simulink model "csws_simulink_model"  (R2021a)
settings: Solver=FixedStepAuto  StartTime=0.0  StopTime=15  RelTol=1e-3
model workspace (MAT data in the model file):
  t = 0
libraries: simulink x1
(part 1 of 2)
settings Model: Creator=Martin  LastModifiedBy=Martin
settings SolverCC: AutoInsertRateTranBlk=on

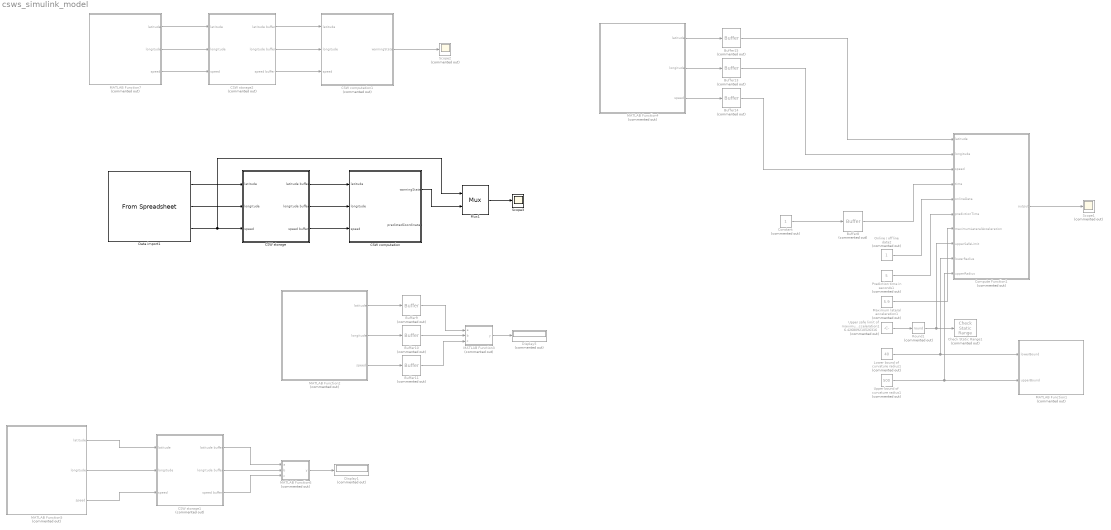
== system csws_simulink_model ==
  Buffer{8..11,13..15} (7 alike) : Buffer  Commented=on  N=3  V=2  ic=-199  OutputFrames=off
  CSW computation : MATLAB Function  TreatAsAtomicUnit=on  mask{timeRate=1, predictionTime=5, maximumLateralAcceleration=5.9, upperSafeLimit=70, lowerRadius=0, upperRadius=5000, visualizeTrajectory=on}
      mask prompts: timeRate "Time frequency of input data (s)"; predictionTime "Prediction time (s)"; maximumLateralAcceleration "Maximum lateral acceleration (m/s^2)"; upperSafeLimit "Safe limit to decrease value of lateral acceleration (0-100%)"; lowerRadius "Lower limit (m)"; upperRadius "Upper limit (m)"; visualizeTrajectory "Visualize trajectory"
  CSW computation1 : MATLAB Function  Commented=on  TreatAsAtomicUnit=on  mask{timeRate=1, predictionTime=5, maximumLateralAcceleration=5.9, upperSafeLimit=70, lowerRadius=0, upperRadius=5000, visualizeTrajectory=on}
      mask prompts: timeRate "Time frequency of input data (s)"; predictionTime "Prediction time (s)"; maximumLateralAcceleration "Maximum lateral acceleration (m/s^2)"; upperSafeLimit "Safe limit to decrease value of lateral acceleration (0-100%)"; lowerRadius "Lower limit (m)"; upperRadius "Upper limit (m)"; visualizeTrajectory "Visualize trajectory"
  CSW storage : Subsystem
  CSW storage1 : Subsystem  Commented=on
  CSW storage2 : Subsystem  Commented=on
  Check Static Range1 : simulink/Model Verification/Check  Static Range  Description=0 <= u <= 100  Commented=on  max=100  max_included=on  min=0  min_included=on  enabled=on  stopWhenAssertionFail=on  export=off  icon=graphic
      settings: SourceProductBaseCode=SL
  Compute Function1 : MATLAB Function  Commented=on  TreatAsAtomicUnit=on
  Constant : Constant  Commented=on
  Data import1 : FromSpreadsheet  FileName=C:\Users\Martin\MATLAB\Projects\curve-speed-warning-system\src\exampleData2.xlsx  SheetName=Hárok1  Range=A1:C11  TreatFirstColumnAs=Data  SampleTime=-1  OutputAfterLastPoint=Ground value
  Display1 : Display  Commented=on
  Display5 : Display  Commented=on
  Lower bound of curvature radius1 : Constant  Commented=on  Value=40
  MATLAB Function1 : MATLAB Function  Commented=on  TreatAsAtomicUnit=on
  MATLAB Function2 : MATLAB Function  Commented=on  TreatAsAtomicUnit=on  mask{inputPort=15}
      mask prompts: inputPort "Serial port - COM"
  MATLAB Function3 : MATLAB Function  Commented=on  TreatAsAtomicUnit=on
  MATLAB Function4 : MATLAB Function  Commented=on  TreatAsAtomicUnit=on
  MATLAB Function5 : MATLAB Function  Commented=on  TreatAsAtomicUnit=on  mask{inputPort=15}
      mask prompts: inputPort "Serial port - COM"
  MATLAB Function6 : MATLAB Function  Commented=on  TreatAsAtomicUnit=on
  MATLAB Function7 : MATLAB Function  Commented=on  TreatAsAtomicUnit=on  mask{inputPort=15}
      mask prompts: inputPort "Serial port - COM"
  Maximum lateral acceleration1 : Constant  Commented=on  Value=5.9
  Mux1 : Mux  Inputs=2
  Online / offline data2 : Constant  Commented=on
  Prediction time in seconds1 : Constant  Commented=on  Value=5
  Round1 : Rounding  Commented=on  Operator=round
  Scope1 : Scope  Commented=on
  Scope2 : Scope  Commented=on
  Scope3 : Scope
  Upper bound of curvature radius1 : Constant  Commented=on  Value=500
  Upper safe limit of maximum lateral acceleration1 : Constant  Commented=on  Value=6.426809210526316
  wires:
  Buffer8/1 -> Compute Function1/4(time)
  Compute Function1/1(output) -> Scope1/1
  Prediction time in seconds1/1 -> Compute Function1/6(predictionTime)
  Upper bound of curvature radius1/1 -> MATLAB Function1/2(upperBound), Compute Function1/10(upperRadius)
  Upper safe limit of maximum lateral acceleration1/1 -> Round1/1
  Lower bound of curvature radius1/1 -> MATLAB Function1/1(lowerBound), Compute Function1/9(lowerRadius)
  Round1/1 -> Check Static Range1/1, Compute Function1/8(upperSafeLimit)
  Maximum lateral acceleration1/1 -> Compute Function1/7(maximumLateralAcceleration)
  Online / offline data2/1 -> Compute Function1/5(onlineData)
  MATLAB Function2/1(latitude) -> Buffer9/1
  MATLAB Function2/2(longitude) -> Buffer10/1
  MATLAB Function2/3(speed) -> Buffer11/1
  Buffer9/1 -> MATLAB Function3/1(a)
  Buffer11/1 -> MATLAB Function3/3(c)
  Buffer10/1 -> MATLAB Function3/2(b)
  MATLAB Function3/1(y) -> Display5/1
  MATLAB Function4/2(longitude) -> Buffer13/1
  MATLAB Function4/3(speed) -> Buffer14/1
  MATLAB Function4/1(latitude) -> Buffer15/1
  Buffer15/1 -> Compute Function1/1(latitude)
  Buffer13/1 -> Compute Function1/2(longitude)
  Buffer14/1 -> Compute Function1/3(speed)
  Constant/1 -> Buffer8/1
  Mux1/1 -> Scope3/1
  Data import1/3 -> Mux1/1, CSW storage/3(speed)
  CSW computation/1(warningState) -> Mux1/2
  Data import1/1 -> CSW storage/1(latitude)
  Data import1/2 -> CSW storage/2(longitude)
  CSW storage/1(latitude buffer) -> CSW computation/1(latitude)
  CSW storage/2(longitude buffer) -> CSW computation/2(longitude)
  CSW storage/3(speed buffer) -> CSW computation/3(speed)
  MATLAB Function6/1(y) -> Display1/1
  MATLAB Function5/2(longitude) -> CSW storage1/2(longitude)
  CSW storage1/2(longitude buffer) -> MATLAB Function6/2(b)
  CSW storage1/1(latitude buffer) -> MATLAB Function6/1(a)
  CSW storage1/3(speed buffer) -> MATLAB Function6/3(c)
  MATLAB Function5/1(latitude) -> CSW storage1/1(latitude)
  MATLAB Function5/3(speed) -> CSW storage1/3(speed)
  MATLAB Function7/3(speed) -> CSW storage2/3(speed)
  MATLAB Function7/2(longitude) -> CSW storage2/2(longitude)
  MATLAB Function7/1(latitude) -> CSW storage2/1(latitude)
  CSW storage2/1(latitude buffer) -> CSW computation1/1(latitude)
  CSW storage2/2(longitude buffer) -> CSW computation1/2(longitude)
  CSW storage2/3(speed buffer) -> CSW computation1/3(speed)
  CSW computation1/1(warningState) -> Scope2/1

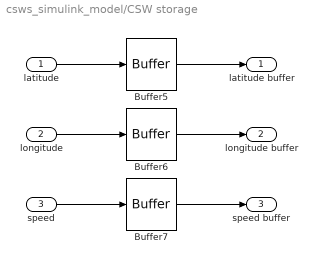
== system csws_simulink_model/CSW storage ==
  latitude : Inport
  longitude : Inport  Port=2
  speed : Inport  Port=3
  Buffer5 : Buffer  N=3  V=2  ic=-199  OutputFrames=off
  Buffer6 : Buffer  N=3  V=2  ic=-199  OutputFrames=off
  Buffer7 : Buffer  N=3  V=2  ic=-199  OutputFrames=off
  latitude buffer : Outport
  longitude buffer : Outport  Port=2
  speed buffer : Outport  Port=3
  wires:
  speed/1 -> Buffer7/1
  Buffer5/1 -> latitude buffer/1
  longitude/1 -> Buffer6/1
  Buffer7/1 -> speed buffer/1
  Buffer6/1 -> longitude buffer/1
  latitude/1 -> Buffer5/1

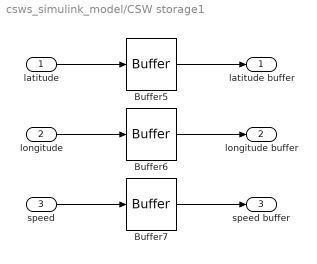
== system csws_simulink_model/CSW storage1 ==
  latitude : Inport
  longitude : Inport  Port=2
  speed : Inport  Port=3
  Buffer5 : Buffer  N=3  V=2  ic=-199  OutputFrames=off
  Buffer6 : Buffer  N=3  V=2  ic=-199  OutputFrames=off
  Buffer7 : Buffer  N=3  V=2  ic=-199  OutputFrames=off
  latitude buffer : Outport
  longitude buffer : Outport  Port=2
  speed buffer : Outport  Port=3
  wires:
  speed/1 -> Buffer7/1
  Buffer5/1 -> latitude buffer/1
  longitude/1 -> Buffer6/1
  Buffer7/1 -> speed buffer/1
  Buffer6/1 -> longitude buffer/1
  latitude/1 -> Buffer5/1

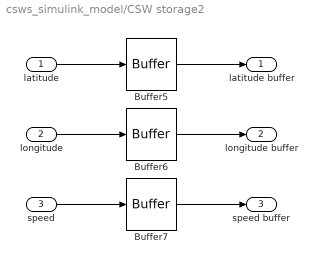
== system csws_simulink_model/CSW storage2 ==
  latitude : Inport
  longitude : Inport  Port=2
  speed : Inport  Port=3
  Buffer5 : Buffer  N=3  V=2  ic=-199  OutputFrames=off
  Buffer6 : Buffer  N=3  V=2  ic=-199  OutputFrames=off
  Buffer7 : Buffer  N=3  V=2  ic=-199  OutputFrames=off
  latitude buffer : Outport
  longitude buffer : Outport  Port=2
  speed buffer : Outport  Port=3
  wires:
  speed/1 -> Buffer7/1
  Buffer5/1 -> latitude buffer/1
  longitude/1 -> Buffer6/1
  Buffer7/1 -> speed buffer/1
  Buffer6/1 -> longitude buffer/1
  latitude/1 -> Buffer5/1

== matlab function csws_simulink_model/CSW computation1 ==
  data: latitude input; longitude input; warningState output; speed input
function warningState = CSW(latitude,longitude,speed)

    coder.extrinsic('plot');
    coder.extrinsic('legend');
    coder.extrinsic('audioread');
    coder.extrinsic('audioplayer');
    coder.extrinsic('serialport');
    coder.extrinsic('readline');
    coder.extrinsic('nmeaParser');
    coder.extrinsic('getfield');
    coder.extrinsic('set_param');
    coder.extrinsic('ceil');
    coder.extrinsic('str2double');
    coder.extrinsic('get_param');
    coder.extrinsic('gcb');
    
    predictionTime = double(0);
    predictionTime = str2double(get_param(gcb,'predictionTime'));
    maximumLateralAcceleration = double(0);
    maximumLateralAcceleration = str2double(get_param(gcb,'maximumLateralAcceleration'));
    upperSafeLimit = double(0);
    upperSafeLimit = str2double(get_param(gcb,'upperSafeLimit'));
    lowerRadius = double(0);
    lowerRadius = str2double(get_param(gcb,'lowerRadius'));
    upperRadius = double(0);
    upperRadius = str2double(get_param(gcb,'upperRadius'));
    timeRate = double(0);
    timeRate = str2double(get_param(gcb,'timeRate'));
    visualizeTrajectory = str2bool(get_param(gcb,'visualizeTrajectory'));
    
    if(upperSafeLimit > 100 || upperSafeLimit < 0)
        error('Invalid value of safe limit, set value in range 0 to 100')
    end
    
    if(lowerRadius < 0 || upperRadius < 0)
        error('Negative value of curvature bound is not supported')
    end

    if(lowerRadius > upperRadius)
        error('Lower bound of curvature radius must be smaller than upper bound')
    end
    
    if(upperSafeLimit > 100 || upperSafeLimit < 0)
        error('Negative value of time frequency is not supported')
    end

%     coder.varsize('output');

    [y, Fs] = audioread('alert.mp3');
    player = audioplayer(y, Fs);
    
    index = 3;

    data = [latitude(:) longitude(:) speed(:)];

    if ismember(-199, data)
        warningState = 0;
        return;
    end

    if (ismember(0, latitude(:)) && ismember(0, longitude(:)) && ismember(0, speed(:)))
        error('Input data contains an invalid zero value/s')
    end

    data = centerDataArray(data);

    allData = [data(index - 2,1) data(index - 2,2) data(index - 2,3); 
        data(index - 1,1) data(index - 1,2) data(index - 1,3); 
        data(index,1) data(index,2) data(index,3)
        ];
    predictedData = [data(index,1) data(index,2) data(index,3)];

    temp_data = [
        data(length(data(:,1))-2,1) data(length(data(:,1))-2,2) data(length(data(:,1))-2,3);
        data(length(data(:,1))-1,1) data(length(data(:,1))-1,2) data(length(data(:,1))-1,3); 
        data(length(data(:,1)),1) data(length(data(:,1)),2) data(length(data(:,1)),3)
        ];

    steps = 0;
    steps = ceil(predictionTime / timeRate);

    for time = 1:steps
        [predictedX, predictedY] = predictCoordinates(temp_data, 3, timeRate);  

        temp_data = [temp_data(2,1) temp_data(2,2) temp_data(2,3);
            temp_data(3,1) temp_data(3,2) temp_data(3,3);
            predictedX predictedY getNextSpeed(temp_data, 3);
            ];

        allData = [allData; [temp_data(3,1) temp_data(3,2) temp_data(3,3)]];
        predictedData = [predictedData; [temp_data(3,1) temp_data(3,2) temp_data(3,3)]];
    end

    allData = computeCurvatureRadiusAndSpeed(allData,maximumLateralAcceleration*((100-upperSafeLimit)/100));

    N = size(allData,1);
    allData = [allData,zeros(N,1)];

    allData = checkCurvatureRadiusAndSpeed(allData, lowerRadius, upperRadius);

    if ismember(1, allData(7,:))
        warningState = 1;
    else
        warningState = 0;
    end

    if(visualizeTrajectory)
        plotOutput(allData, predictedData, timeRate, player);
    end
%     else
% %         set_param('asik','Commented','on')
% %         PORT = "COM15";
%         PORT = serialPort;
%         device = serialport(PORT,9600)
%         pnmea = nmeaParser("MessageIDs", "RMC");
%         
%         record = readline(device);
%         
%         while (isempty(record) || ~startsWith(record,'$GPRMC'))
%             record = readline(device);
%         end        
%         
%         nvm = pnmea(record);
%         Latitude = getfield(nvm,'Latitude');
%         Longitude = getfield(nvm,'Longitude');
%         Speed = getfield(nvm,'GroundSpeed');
%         Time = getfield(nvm,'UTCDateTime');
% %         fldnm = 'Status';
% %         nx2 = nvm.parameters.(fldnm)
% %         latit = output(Latitude)
% %         gpsData = struct('Latitude',output.Latitude,'Longitude',output.Longitude,'Speed',output.GroundSpeed,'Time',output.UTCDateTime,'Status',output.Status);
% 
% 
% %     if (speed(3) > 21)
% %         output = 1
% %     else
% %         output = 0
% %     end
% 
% 
%         warningState = 3
%     end

end

function MyBeep()
    coder.extrinsic('audioplayer');
    coder.extrinsic('play');
    persistent AP
    Play_Data = ([sin(1:.6:400), sin(1:.7:400), sin(1:.4:400)]);
    AP = audioplayer(Play_Data(:), 22050);
    play(AP);
end

function [output]=str2bool(string)
   if strcmp(string,'off')
     output = false;
   else
     output = true;
   end
end

%% plot output prediction trajectory with / without warning

function plotOutput(allData, predictedData, timeRate, player)
    coder.extrinsic('plot');
    coder.extrinsic('legend');
    coder.extrinsic('playblocking');
    coder.extrinsic('play');
    coder.extrinsic('strcat');
    
    x_min = min(allData(:,1)) - 5;
    x_max = max(allData(:,1)) + 5;
    
    x1 =  abs(x_min);
    x2 =  abs(x_max);
    
    result = x1;
    if(x1 < x2)
        result = x2;
    end
    
    y_min = min(allData(:,2)) - 5;
    y_max = max(allData(:,2)) + 5;
    
    plot(allData(:,1), allData(:,2), 'b-o', 'DisplayName','referenced coordinates')
    xlim([-result result])
    ylim([y_min y_max])
    hold on
    plot(predictedData(:,1), predictedData(:,2), 'g-o', 'DisplayName','predicted coordinates')
    plot(predictedData(1,1), predictedData(1,2), 'k-o', 'DisplayName','actual position')
    title(sprintf('point frequency is %.1f second/s',timeRate));
    legend('referenced coordinates','predicted coordinates','actual position')
    
    if ismember(1, allData(:,7))
        set(gca, 'Color',[1 0 0])
%         MyBeep()
%         playblocking(player); 
    else
        set(gca, 'Color',[1 1 1])
    end

    hold off
end

%% compute radius of curvature and recommended speed

function [predictedData] = computeCurvatureRadiusAndSpeed(predictedData,safeLimitOfLateralAcceleration)
    Alateral_max = safeLimitOfLateralAcceleration;

    [pathdistance,R,~] = curvature([predictedData(:,1) predictedData(:,2)]);
    predictedData = [predictedData pathdistance R];
    predictedData = [predictedData sqrt(predictedData(:, 5) * Alateral_max)];
end


%% reference to: https://uk.mathworks.com/matlabcentral/fileexchange/69452-curvature-of-a-1d-curve-in-a-2d-or-3d-space 

function [L,R,k] = curvature(input)
% Radius of curvature and curvature vector for 2D or 3D curve
%  [L,R,k] = curvature(X)
%   X:   2 or 3 column array of x, y (and possibly z) coordiates
%   L:   Cumulative arc length
%   R:   Radius of curvature
%   k:   Curvature vector
% The scalar curvature value is 1./R
% Version 2.6: Calculates end point values for closed curve
%   fefefe = X

  coder.varsize('X');
  coder.varsize('L');
  coder.varsize('R');
  coder.varsize('k');
  X = input;

  N = size(X,1);
  dims = size(X,2);
  if dims == 2
    X = [X,zeros(N,1)];  % Use 3D expressions for 2D as well
  end
  L = zeros(N,1);
  R = NaN(N,1);
  k = NaN(N,3);
  for i = 2:N-1
    [R(i),~,k(i,:)] = circumcenter(X(i,:)',X(i-1,:)',X(i+1,:)');
    L(i) = L(i-1)+norm(X(i,:)-X(i-1,:));
  end
  if norm(X(1,:)-X(end,:)) < 1e-10 % Closed curve. 
    [R(1),~,k(1,:)] = circumcenter(X(end-1,:)',X(1,:)',X(2,:)');
    R(end) = R(1);
    k(end,:) = k(1,:);
    L(end) = L(end-1) + norm(X(end,:)-X(end-1,:));
  end
  i = N;
  L(i) = L(i-1)+norm(X(i,:)-X(i-1,:));
  if dims == 2
    k = k(:,1:2);
  end
end

%% reference to: https://uk.mathworks.com/matlabcentral/fileexchange/69452-curvature-of-a-1d-curve-in-a-2d-or-3d-space 

function [R,M,k] = circumcenter(A,B,C)
% Center and radius of the circumscribed circle for the triangle ABC
%  A,B,C  3D coordinate vectors for the triangle corners
%  R      Radius
%  M      3D coordinate vector for the center
%  k      Vector of length 1/R in the direction from A towards M
%         (Curvature vector)
  D = cross(B-A,C-A);
  b = norm(A-C);
  c = norm(A-B);
  if nargout == 1
    a = norm(B-C);     % slightly faster if only R is required
    R = a*b*c/2/norm(D);
    if norm(D) == 0
      R = Inf;
    end
    return
  end
  E = cross(D,B-A);
  F = cross(D,C-A); 
  G = (b^2*E-c^2*F)/norm(D)^2/2;
  M = A + G;
  R = norm(G);  % Radius of curvature
  if R == 0
    k = G;
  elseif norm(D) == 0
    R = Inf;
    k = D;
  else
    k = G'/R^2;   % Curvature vector
  end
end

%% check if radius of curvature is valid and actual speed is higher than recommended

function [predictedData] = checkCurvatureRadiusAndSpeed(predictedData,lowerRadius,upperRadius)
    Rmin = lowerRadius;
    Rmax = upperRadius;
    
    for k=1:size(predictedData,1)
        if predictedData(k,5) < Rmin || predictedData(k,5) > Rmax
            predictedData(k,7) = 0;
        else
            if predictedData(k,3) > predictedData(k,6)
                predictedData(k,7) = 1;
            else
                predictedData(k,7) = 0;
            end
        end
    end
end

%% compute angle between coordinates

function next_angle = computeCoordinateAngle(data, index, time)
    prev_angle = atan2( (data(index - 1,2) - data(index - 2,2)) , (data(index - 1,1) - data(index - 2,1)));
    act_angle = atan2( (data(index,2) - data(index - 1,2)) , (data(index,1) - data(index - 1,1)));
    
    next_angle = act_angle + time*(act_angle - prev_angle);
end

%% convert latitude, longitude to cartesian coordinate system

function [data] = centerDataArray(data)
    centered_point = [0 1];
    
    data = convertDataArray(data);

    angle = atan2(centered_point(1,2) - data(3,2), centered_point(1,1) - data(3,1)) - atan2(data(2,2) - data(3,2), data(2,1) - data(3,1));
    result = deg2rad(180) - angle;

    x2 = data(2,1) * cos(result) + data(2,2) * sin(result);
    y2 = data(2,1) * -sin(result) + data(2,2) *  cos(result);

    x1 = data(1,1) * cos(result) + data(1,2) * sin(result);
    y1 = data(1,1) * -sin(result) + data(1,2) *  cos(result);

    centeredData = [x1 y1; x2 y2; data(3,1) data(3,2)];
    data(:,1) = centeredData(:,1);
    data(:,2) = centeredData(:,2);
end

%% convert latitude, longitude to cartesian coordinate system

function [data] = convertDataArray(data)
    coder.extrinsic('latlon2local');
    [xCoordinate, yCoordinate] = latlon2local(data(:,1), data(:,2), 0, [data(3,1), data(3,2), 0]);
    data = [xCoordinate yCoordinate data(:,3)];
end

%% get speed of last referenced point for predicted points

function [nextspeed] = getNextSpeed(data, index)
    nextspeed = data(index,3);
    if nextspeed < 0
        nextspeed = 0;
    end
end

%% insert GPS data to data structure

function [predictedX,predictedY] = predictCoordinates(data, index, time)
    speed = getNextSpeed(data, index);
    next_angle = computeCoordinateAngle(data, index, time);

    predictedX = predictCoordinateX(data, index, next_angle, time, speed);
    predictedY = predictCoordinateY(data, index, next_angle, time, speed);
end

%% predict x coordinate

function predictedX = predictCoordinateX(data, index, angle, time, speed)
    predictedX = data(index,1) + speed * time * cos(angle);
end

%% predict y coordinate

function predictedY = predictCoordinateY(data, index, angle, time, speed)
    predictedY = data(index,2) + speed * time * sin(angle);
end

== matlab function csws_simulink_model/MATLAB Function7 ==
  data: latitude output; longitude output; speed output
function [latitude, longitude, speed] = GPSDataReceiver

coder.extrinsic('serialport');
coder.extrinsic('readline');
coder.extrinsic('nmeaParser');
coder.extrinsic('getfield');
coder.extrinsic('set_param');
coder.extrinsic('strings');
coder.extrinsic('strrep');

coder.extrinsic('str2double');
coder.extrinsic('get_param');
coder.extrinsic('gcb');
coder.extrinsic('append');

inputPort = get_param(gcb,'inputPort');

% coder.varsize('latitude')
% coder.varsize('longitude')
% coder.varsize('speed')
% coder.varsize('time')
latitude=zeros(1,1);
longitude=zeros(1,1);
speed=zeros(1,1);
% time=strings(1);

        PORT = append("COM",inputPort);
        device = serialport(PORT,9600);
        pnmea = nmeaParser("MessageIDs", "RMC");
        
        record = readline(device);
        
        while (isempty(record) || ~startsWith(record,'$GPRMC'))
            record = readline(device);
        end        
        
        nvm = pnmea(record);
        latitude = getfield(nvm,'Latitude');
        longitude = getfield(nvm,'Longitude');
        speed = getfield(nvm,'GroundSpeed');
        
        latitude = strrep(latitude,'.',',');
        longitude = strrep(longitude,'.',',');
        speed = strrep(speed,'.',',');
%         time = getfield(nvm,'UTCDateTime');

%         a = size(latitude)
%         b = size(fx)  
%         x = length(latitude)
%         b = size(latitude(1))
% [latitude, longitude, speed, time]
% y = latitude
% y = latitude
f = latitude

== matlab function csws_simulink_model/CSW computation ==
  data: latitude input; longitude input; warningState output; speed input; predictedCoordinates output
function [warningState, predictedCoordinates] = CSW(latitude,longitude,speed)

    coder.extrinsic('plot');
    coder.extrinsic('legend');
    coder.extrinsic('audioread');
    coder.extrinsic('audioplayer');
    coder.extrinsic('serialport');
    coder.extrinsic('readline');
    coder.extrinsic('nmeaParser');
    coder.extrinsic('getfield');
    coder.extrinsic('set_param');
    coder.extrinsic('ceil');
    coder.extrinsic('str2double');
    coder.extrinsic('get_param');
    coder.extrinsic('gcb');
    
    coder.varsize('predictedCoordinates');
    
    predictionTime = double(0);
    predictionTime = str2double(get_param(gcb,'predictionTime'));
    maximumLateralAcceleration = double(0);
    maximumLateralAcceleration = str2double(get_param(gcb,'maximumLateralAcceleration'));
    upperSafeLimit = double(0);
    upperSafeLimit = str2double(get_param(gcb,'upperSafeLimit'));
    lowerRadius = double(0);
    lowerRadius = str2double(get_param(gcb,'lowerRadius'));
    upperRadius = double(0);
    upperRadius = str2double(get_param(gcb,'upperRadius'));
    timeRate = double(0);
    timeRate = str2double(get_param(gcb,'timeRate'));
    visualizeTrajectory = str2bool(get_param(gcb,'visualizeTrajectory'));
    
    if(upperSafeLimit > 100 || upperSafeLimit < 0)
        error('Invalid value of safe limit, set value in range 0 to 100')
    end
    
    if(lowerRadius < 0 || upperRadius < 0)
        error('Negative value of curvature bound is not supported')
    end

    if(lowerRadius > upperRadius)
        error('Lower bound of curvature radius must be smaller than upper bound')
    end
    
    if(upperSafeLimit > 100 || upperSafeLimit < 0)
        error('Negative value of time frequency is not supported')
    end

%     coder.varsize('output');

    [y, Fs] = audioread('alert.mp3');
    player = audioplayer(y, Fs);
    
    index = 3;

    data = [latitude(:) longitude(:) speed(:)];

    if ismember(-199, data)
        warningState = 0;
        predictedCoordinates = [];
        return;
    end

    if (ismember(0, latitude(:)) && ismember(0, longitude(:)) && ismember(0, speed(:)))
        error('Input data contains an invalid zero value/s')
    end

    data = centerDataArray(data);

    allData = [data(index - 2,1) data(index - 2,2) data(index - 2,3); 
        data(index - 1,1) data(index - 1,2) data(index - 1,3); 
        data(index,1) data(index,2) data(index,3)
        ];
    predictedData = [data(index,1) data(index,2) data(index,3)];

    temp_data = [
        data(length(data(:,1))-2,1) data(length(data(:,1))-2,2) data(length(data(:,1))-2,3);
        data(length(data(:,1))-1,1) data(length(data(:,1))-1,2) data(length(data(:,1))-1,3); 
        data(length(data(:,1)),1) data(length(data(:,1)),2) data(length(data(:,1)),3)
        ];

    steps = 0;
    steps = ceil(predictionTime / timeRate);

    for time = 1:steps
        [predictedX, predictedY] = predictCoordinates(temp_data, 3, timeRate);  

        temp_data = [temp_data(2,1) temp_data(2,2) temp_data(2,3);
            temp_data(3,1) temp_data(3,2) temp_data(3,3);
            predictedX predictedY getNextSpeed(temp_data, 3);
            ];

        allData = [allData; [temp_data(3,1) temp_data(3,2) temp_data(3,3)]];
        predictedData = [predictedData; [temp_data(3,1) temp_data(3,2) temp_data(3,3)]];
    end

    allData = computeCurvatureRadiusAndSpeed(allData,maximumLateralAcceleration*((100-upperSafeLimit)/100));

    N = size(allData,1);
    allData = [allData,zeros(N,1)];

    allData = checkCurvatureRadiusAndSpeed(allData, lowerRadius, upperRadius);

    predictedCoordinates = [predictedData(:,1), predictedData(:,2)];

    if ismember(1, allData(7,:))
        warningState = 1;
    else
        warningState = 0;
    end

    if(visualizeTrajectory)
        plotOutput(allData, predictedData, timeRate, player);
    end
%     else
% %         set_param('asik','Commented','on')
% %         PORT = "COM15";
%         PORT = serialPort;
%         device = serialport(PORT,9600)
%         pnmea = nmeaParser("MessageIDs", "RMC");
%         
%         record = readline(device);
%         
%         while (isempty(record) || ~startsWith(record,'$GPRMC'))
%             record = readline(device);
%         end        
%         
%         nvm = pnmea(record);
%         Latitude = getfield(nvm,'Latitude');
%         Longitude = getfield(nvm,'Longitude');
%         Speed = getfield(nvm,'GroundSpeed');
%         Time = getfield(nvm,'UTCDateTime');
% %         fldnm = 'Status';
% %         nx2 = nvm.parameters.(fldnm)
% %         latit = output(Latitude)
% %         gpsData = struct('Latitude',output.Latitude,'Longitude',output.Longitude,'Speed',output.GroundSpeed,'Time',output.UTCDateTime,'Status',output.Status);
% 
% 
% %     if (speed(3) > 21)
% %         output = 1
% %     else
% %         output = 0
% %     end
% 
% 
%         warningState = 3
%     end

end

function MyBeep()
    coder.extrinsic('audioplayer');
    coder.extrinsic('play');
    persistent AP
    Play_Data = ([sin(1:.6:400), sin(1:.7:400), sin(1:.4:400)]);
    AP = audioplayer(Play_Data(:), 22050);
    play(AP);
end

function [output]=str2bool(string)
   if strcmp(string,'off')
     output = false;
   else
     output = true;
   end
end

%% plot output prediction trajectory with / without warning

function plotOutput(allData, predictedData, timeRate, player)
    coder.extrinsic('plot');
    coder.extrinsic('legend');
    coder.extrinsic('playblocking');
    coder.extrinsic('play');
    coder.extrinsic('strcat');
    
    x_min = min(allData(:,1)) - 5;
    x_max = max(allData(:,1)) + 5;
    
    x1 =  abs(x_min);
    x2 =  abs(x_max);
    
    result = x1;
    if(x1 < x2)
        result = x2;
    end
    
    y_min = min(allData(:,2)) - 5;
    y_max = max(allData(:,2)) + 5;
    
    plot(allData(:,1), allData(:,2), 'b-o', 'DisplayName','referenced coordinates')
    xlim([-result result])
    ylim([y_min y_max])
    hold on
    plot(predictedData(:,1), predictedData(:,2), 'g-o', 'DisplayName','predicted coordinates')
    plot(predictedData(1,1), predictedData(1,2), 'k-o', 'DisplayName','actual position')
    title(sprintf('point frequency is %.1f second/s',timeRate));
    legend('referenced coordinates','predicted coordinates','actual position')
    
    if ismember(1, allData(:,7))
        set(gca, 'Color',[1 0 0])
%         MyBeep()
%         playblocking(player); 
    else
        set(gca, 'Color',[1 1 1])
    end

    hold off
end

%% compute radius of curvature and recommended speed

function [predictedData] = computeCurvatureRadiusAndSpeed(predictedData,safeLimitOfLateralAcceleration)
    Alateral_max = safeLimitOfLateralAcceleration;

    [pathdistance,R,~] = curvature([predictedData(:,1) predictedData(:,2)]);
    predictedData = [predictedData pathdistance R];
    predictedData = [predictedData sqrt(predictedData(:, 5) * Alateral_max)];
end


%% reference to: https://uk.mathworks.com/matlabcentral/fileexchange/69452-curvature-of-a-1d-curve-in-a-2d-or-3d-space 

function [L,R,k] = curvature(input)
% Radius of curvature and curvature vector for 2D or 3D curve
%  [L,R,k] = curvature(X)
%   X:   2 or 3 column array of x, y (and possibly z) coordiates
%   L:   Cumulative arc length
%   R:   Radius of curvature
%   k:   Curvature vector
% The scalar curvature value is 1./R
% Version 2.6: Calculates end point values for closed curve
%   fefefe = X

  coder.varsize('X');
  coder.varsize('L');
  coder.varsize('R');
  coder.varsize('k');
  X = input;

  N = size(X,1);
  dims = size(X,2);
  if dims == 2
    X = [X,zeros(N,1)];  % Use 3D expressions for 2D as well
  end
  L = zeros(N,1);
  R = NaN(N,1);
  k = NaN(N,3);
  for i = 2:N-1
    [R(i),~,k(i,:)] = circumcenter(X(i,:)',X(i-1,:)',X(i+1,:)');
    L(i) = L(i-1)+norm(X(i,:)-X(i-1,:));
  end
  if norm(X(1,:)-X(end,:)) < 1e-10 % Closed curve. 
    [R(1),~,k(1,:)] = circumcenter(X(end-1,:)',X(1,:)',X(2,:)');
    R(end) = R(1);
    k(end,:) = k(1,:);
    L(end) = L(end-1) + norm(X(end,:)-X(end-1,:));
  end
  i = N;
  L(i) = L(i-1)+norm(X(i,:)-X(i-1,:));
  if dims == 2
    k = k(:,1:2);
  end
end

%% reference to: https://uk.mathworks.com/matlabcentral/fileexchange/69452-curvature-of-a-1d-curve-in-a-2d-or-3d-space 

function [R,M,k] = circumcenter(A,B,C)
% Center and radius of the circumscribed circle for the triangle ABC
%  A,B,C  3D coordinate vectors for the triangle corners
%  R      Radius
%  M      3D coordinate vector for the center
%  k      Vector of length 1/R in the direction from A towards M
%         (Curvature vector)
  D = cross(B-A,C-A);
  b = norm(A-C);
  c = norm(A-B);
  if nargout == 1
    a = norm(B-C);     % slightly faster if only R is required
    R = a*b*c/2/norm(D);
    if norm(D) == 0
      R = Inf;
    end
    return
  end
  E = cross(D,B-A);
  F = cross(D,C-A); 
  G = (b^2*E-c^2*F)/norm(D)^2/2;
  M = A + G;
  R = norm(G);  % Radius of curvature
  if R == 0
    k = G;
  elseif norm(D) == 0
    R = Inf;
    k = D;
  else
    k = G'/R^2;   % Curvature vector
  end
end

%% check if radius of curvature is valid and actual speed is higher than recommended

function [predictedData] = checkCurvatureRadiusAndSpeed(predictedData,lowerRadius,upperRadius)
    Rmin = lowerRadius;
    Rmax = upperRadius;
    
    for k=1:size(predictedData,1)
        if predictedData(k,5) < Rmin || predictedData(k,5) > Rmax
            predictedData(k,7) = 0;
        else
            if predictedData(k,3) > predictedData(k,6)
                predictedData(k,7) = 1;
            else
                predictedData(k,7) = 0;
            end
        end
    end
end

%% compute angle between coordinates

function next_angle = computeCoordinateAngle(data, index, time)
    prev_angle = atan2( (data(index - 1,2) - data(index - 2,2)) , (data(index - 1,1) - data(index - 2,1)));
    act_angle = atan2( (data(index,2) - data(index - 1,2)) , (data(index,1) - data(index - 1,1)));
    
    next_angle = act_angle + time*(act_angle - prev_angle);
end

%% convert latitude, longitude to cartesian coordinate system

function [data] = centerDataArray(data)
    centered_point = [0 1];
    
    data = convertDataArray(data);

    angle = atan2(centered_point(1,2) - data(3,2), centered_point(1,1) - data(3,1)) - atan2(data(2,2) - data(3,2), data(2,1) - data(3,1));
    result = deg2rad(180) - angle;

    x2 = data(2,1) * cos(result) + data(2,2) * sin(result);
    y2 = data(2,1) * -sin(result) + data(2,2) *  cos(result);

    x1 = data(1,1) * cos(result) + data(1,2) * sin(result);
    y1 = data(1,1) * -sin(result) + data(1,2) *  cos(result);

    centeredData = [x1 y1; x2 y2; data(3,1) data(3,2)];
    data(:,1) = centeredData(:,1);
    data(:,2) = centeredData(:,2);
end

%% convert latitude, longitude to cartesian coordinate system

function [data] = convertDataArray(data)
    coder.extrinsic('latlon2local');
    [xCoordinate, yCoordinate] = latlon2local(data(:,1), data(:,2), 0, [data(3,1), data(3,2), 0]);
    data = [xCoordinate yCoordinate data(:,3)];
end

%% get speed of last referenced point for predicted points

function [nextspeed] = getNextSpeed(data, index)
    nextspeed = data(index,3);
    if nextspeed < 0
        nextspeed = 0;
    end
end

%% insert GPS data to data structure

function [predictedX,predictedY] = predictCoordinates(data, index, time)
    speed = getNextSpeed(data, index);
    next_angle = computeCoordinateAngle(data, index, time);

    predictedX = predictCoordinateX(data, index, next_angle, time, speed);
    predictedY = predictCoordinateY(data, index, next_angle, time, speed);
end

%% predict x coordinate

function predictedX = predictCoordinateX(data, index, angle, time, speed)
    predictedX = data(index,1) + speed * time * cos(angle);
end

%% predict y coordinate

function predictedY = predictCoordinateY(data, index, angle, time, speed)
    predictedY = data(index,2) + speed * time * sin(angle);
end
